simulink model "s_carro_pend"  (R2014a)
settings: Solver=ode3  StartTime=0.0  StopTime=inf  FixedStep=h  RelTol=1e-3
values from neighbouring files (symbols this model uses):
  g = 9.81    [Constantes.m]
  l = 0.641    [Constantes.m]
  m = 0.23    [Constantes.m]
  M = 0.57    [Constantes.m]
undefined symbols (not defined in the file or in its folder): br, bt
libraries: vrlib x3, fuzblock x1
settings Model: Creator=Jovani  LastModifiedBy=Lalo
settings OptimizationCC: SimCompilerOptimization=off
settings DebuggingCC: UnderspecifiedInitializationDetection=Classic  FrameProcessingCompatibilityMsg=error  StateNameClashWarn=warning
settings HardwareCC: ProdBitPerLong=64  ProdBitPerPointer=64  ProdIntDivRoundTo=Zero  ProdEndianess=LittleEndian  ProdWordSize=64  ProdHWDeviceType=Intel->x86-64  TargetBitPerLong=64  TargetBitPerPointer=64  TargetIntDivRoundTo=Zero  TargetEndianess=LittleEndian  TargetWordSize=64  TargetHWDeviceType=Intel->x86-64
settings RTWCC: SystemTargetFile=sldrt.tlc  TemplateMakefile=sldrt.tmf  Description=Simulink Desktop Real-Time  RTWCompilerOptimization=on
settings CodeAppCC: MaxIdLength=95
settings SimulinkDesktopRealTimeCC: TargetPreCompLibLocation=C:\Program Files\MATLAB\R2016a\toolbox\sldrt\lib\win64  TargetLangStandard=C89/C90 (ANSI)  SupportVariableSizeSignals=off
settings ConfigComp: CovMetricSettings=dw  CovHtmlReporting=on  CovSaveCumulativeToWorkspaceVar=on  CovSaveSingleToWorkspaceVar=on  CovModelRefEnable=Off  CovExternalEMLEnable=off

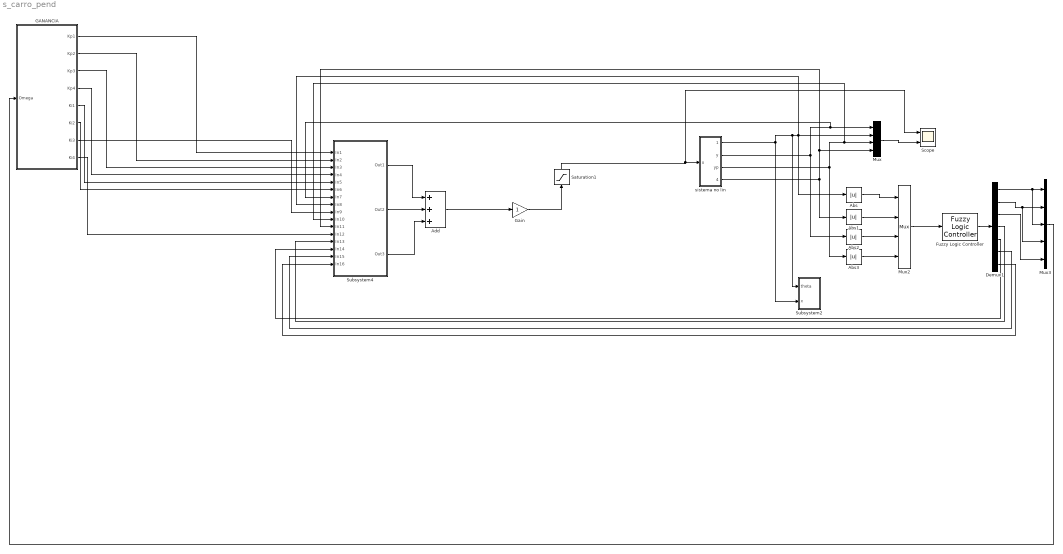
== system s_carro_pend ==
  Abs{,1..3} (4 alike) : Abs
  Add : Sum  Inputs=+++
  Demux1 : Demux  Outputs=7
  Fuzzy Logic Controller : fuzblock/Fuzzy Logic  Controller  fis=pi_2
  GANANCIA : Subsystem
  Gain : Gain
  Mux : Mux
  Mux2 : Mux
  Mux3 : Mux  Inputs=5
  Saturation1 : Saturate  UpperLimit=7.5  LowerLimit=-7.5
  Scope : Scope  NumInputPorts=2
      settings: YMin=-5~-5  YMax=5~5
  Subsystem2 : Subsystem
  Subsystem4 : Subsystem
  sistema no lin : Subsystem
  wires:
  Mux/1 -> Scope/2
  Gain/1 -> Saturation1/1
  Add/1 -> Gain/1
  sistema no lin/2(y) -> Abs2/1, Subsystem4/7(In7), Mux/1
  sistema no lin/3(yp) -> Abs3/1, Subsystem4/10(In10), Mux/3
  sistema no lin/1(theta) -> Subsystem2/2(x), Subsystem2/1(theta), Abs/1, Subsystem4/8(In8), Mux/2
  sistema no lin/4(thetap) -> Abs1/1, Subsystem4/11(In11), Mux/4
  Abs/1 -> Mux2/1
  Abs1/1 -> Mux2/2
  Abs2/1 -> Mux2/3
  Abs3/1 -> Mux2/4
  Mux2/1 -> Fuzzy Logic Controller/1
  Fuzzy Logic Controller/1 -> Demux1/1
  Demux1/1 -> Mux3/3, Mux3/1
  Demux1/2 -> Mux3/4, Mux3/2
  Demux1/3 -> Mux3/5
  Mux3/1 -> GANANCIA/1(Omega)
  Saturation1/1 -> Scope/1, sistema no lin/1("u ")
  ? -> ?
  GANANCIA/1(Kp1) -> Subsystem4/1(In1)
  GANANCIA/2(Kp2) -> Subsystem4/2(In2)
  GANANCIA/3("Kp3 ") -> Subsystem4/3(In3)
  GANANCIA/4(Kp4) -> Subsystem4/4(In4)
  GANANCIA/5("Ki1 ") -> Subsystem4/5(In5)
  GANANCIA/6("Ki2 ") -> Subsystem4/6(In6)
  GANANCIA/7("Ki3 ") -> Subsystem4/9(In9)
  GANANCIA/8("Ki4 ") -> Subsystem4/12(In12)
  Demux1/4 -> Subsystem4/13(In13)
  Demux1/5 -> Subsystem4/14(In14)
  Demux1/6 -> Subsystem4/15(In15)
  Demux1/7 -> Subsystem4/16(In16)
  Subsystem4/1(Out1) -> Add/1
  Subsystem4/2(Out2) -> Add/2
  Subsystem4/3(Out3) -> Add/3

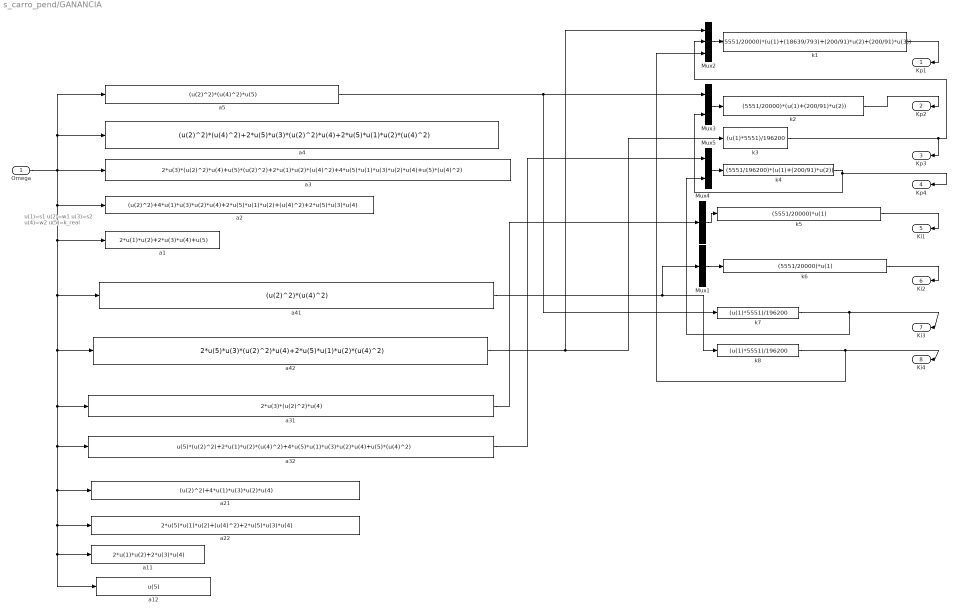
== system s_carro_pend/GANANCIA ==
  note: u(1)=s1
      | u(2)=w1
      | u(3)=s2
      | u(4)=w2
      | u(5)=k_real
  Omega : Inport
  Mux1 : Mux  Inputs=1
  Mux2 : Mux  Inputs=3
  Mux3 : Mux  Inputs=2
  Mux4 : Mux  Inputs=1
  Mux5 : Mux  Inputs=2
  "a1 " : Fcn  Expr=2*u(1)*u(2)+2*u(3)*u(4)+u(5)
  "a11 " : Fcn  Expr=2*u(1)*u(2)+2*u(3)*u(4)
  a12 : Fcn  Expr=u(5)
  "a2 " : Fcn  Expr=(u(2)^2)+4*u(1)*u(3)*u(2)*u(4)+2*u(5)*u(1)*u(2)+(u(4)^2)+2*u(5)*u(3)*u(4)
  "a21 " : Fcn  Expr=(u(2)^2)+4*u(1)*u(3)*u(2)*u(4)
  "a22 " : Fcn  Expr=2*u(5)*u(1)*u(2)+(u(4)^2)+2*u(5)*u(3)*u(4)
  a3 : Fcn  Expr=2*u(3)*(u(2)^2)*u(4)+u(5)*(u(2)^2)+2*u(1)*u(2)*(u(4)^2)+4*u(5)*u(1)*u(3)*u(2)*u(4)+u(5)*(u(4)^2)
  a31 : Fcn  Expr=2*u(3)*(u(2)^2)*u(4)
  a32 : Fcn  Expr=u(5)*(u(2)^2)+2*u(1)*u(2)*(u(4)^2)+4*u(5)*u(1)*u(3)*u(2)*u(4)+u(5)*(u(4)^2)
  a4 : Fcn  Expr=(u(2)^2)*(u(4)^2)+2*u(5)*u(3)*(u(2)^2)*u(4)+2*u(5)*u(1)*u(2)*(u(4)^2)
  a41 : Fcn  Expr=(u(2)^2)*(u(4)^2)
  a42 : Fcn  Expr=2*u(5)*u(3)*(u(2)^2)*u(4)+2*u(5)*u(1)*u(2)*(u(4)^2)
  a5 : Fcn  Expr=(u(2)^2)*(u(4)^2)*u(5)
  k1 : Fcn  Expr=(5551/20000)*(u(1)+(18639/793)+(200/91)*u(2)+(200/91)*u(3))
  k2 : Fcn  Expr=(5551/20000)*(u(1)+(200/91)*u(2))
  k3 : Fcn  Expr=(u(1)*5551)/196200
  k4 : Fcn  Expr=(5551/196200)*(u(1)+(200/91)*u(2))
  "k5 " : Fcn  Expr=(5551/20000)*u(1)
  "k6 " : Fcn  Expr=(5551/20000)*u(1)
  k7 : Fcn  Expr=(u(1)*5551)/196200
  k8 : Fcn  Expr=(u(1)*5551)/196200
  Kp1 : Outport
  Kp2 : Outport  Port=2
  "Kp3 " : Outport  Port=3
  Kp4 : Outport  Port=4
  "Ki1 " : Outport  Port=5
  "Ki2 " : Outport  Port=6
  "Ki3 " : Outport  Port=7
  "Ki4 " : Outport  Port=8
  wires:
  a32/1 -> Mux5/1
  Mux5/1 -> k4/1
  Mux1/1 -> "k6 "/1
  "k6 "/1 -> "Ki2 "/1
  a31/1 -> Mux4/1
  a41/1 -> k8/1, Mux1/1
  a42/1 -> k3/1, Mux2/1
  k2/1 -> Kp2/1
  k1/1 -> Kp1/1
  Mux3/1 -> k2/1
  Mux2/1 -> k1/1
  k4/1 -> Kp4/1, Mux3/2
  "k5 "/1 -> "Ki1 "/1
  k8/1 -> "Ki4 "/1, Mux2/3
  k3/1 -> "Kp3 "/1, Mux2/2
  a5/1 -> Mux3/1, k7/1
  k7/1 -> "Ki3 "/1, Mux5/2
  Omega/1 -> a4/1, a5/1, a3/1, "a2 "/1, "a1 "/1, a41/1, a42/1, a31/1, a32/1, "a21 "/1, "a22 "/1, "a11 "/1, a12/1
  Mux4/1 -> "k5 "/1

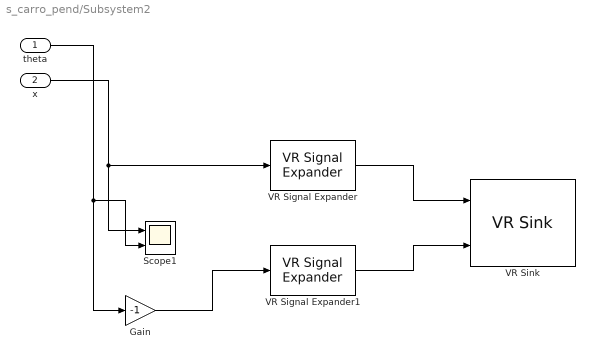
== system s_carro_pend/Subsystem2 ==
  theta : Inport
  x : Inport  Port=2
  Gain : Gain  Gain=-1
  Scope1 : Scope  NumInputPorts=2
      settings: YMin=3.51931e+09~-5.59031e+09  YMax=3.51951e+09~-5.5902e+09
  VR Signal Expander : vrlib/VR Signal Expander  outwidth=3  outidx=[1]
  VR Signal Expander1 : vrlib/VR Signal Expander  outwidth=4  outidx=[4]
  VR Sink : vrlib/VR Sink  InstantiateOnLoad=on  SampleTime=0.1  ViewEnable=on  RemoteChange=off  RemoteView=off  FieldsWritten=Carro.rotation.4.1.1.double#Carro.translation.3.1.1.double  WorldFileName=C:\Users\Lalo\Desktop\MC Automatizacion\Segundo Semestre\Control Int\Carro_pendulo\pendulo_invertido.wrl  AutoView=off  VideoDimensions=[]  AllowVariableSize=off
  wires:
  Gain/1 -> VR Signal Expander1/1
  x/1 -> Scope1/1, VR Signal Expander/1
  theta/1 -> Gain/1, Scope1/2
  VR Signal Expander/1 -> VR Sink/1
  VR Signal Expander1/1 -> VR Sink/2

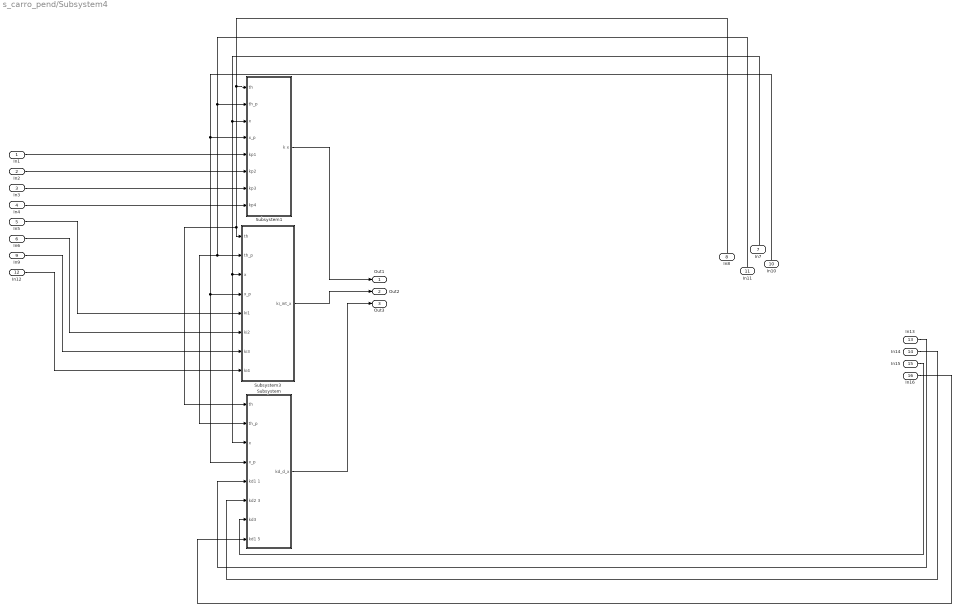
== system s_carro_pend/Subsystem4 ==
  In1 : Inport
  In2 : Inport  Port=2
  In3 : Inport  Port=3
  In4 : Inport  Port=4
  In5 : Inport  Port=5
  In6 : Inport  Port=6
  In7 : Inport  Port=7
  In8 : Inport  Port=8
  In9 : Inport  Port=9
  In10 : Inport  Port=10
  In11 : Inport  Port=11
  In12 : Inport  Port=12
  In13 : Inport  Port=13
  In14 : Inport  Port=14
  In15 : Inport  Port=15
  In16 : Inport  Port=16
  Subsystem : Subsystem
  Subsystem1 : Subsystem
  Subsystem3 : Subsystem
  Out1 : Outport
  Out2 : Outport  Port=2
  Out3 : Outport  Port=3
  wires:
  In1/1 -> Subsystem1/5("kp1 ")
  In2/1 -> Subsystem1/6(kp2)
  In3/1 -> Subsystem1/7(kp3)
  In4/1 -> Subsystem1/8(kp4)
  In5/1 -> Subsystem3/5(ki1)
  In6/1 -> Subsystem3/6(ki2)
  In9/1 -> Subsystem3/7(ki3)
  In12/1 -> Subsystem3/8(ki4)
  Subsystem1/1(k x) -> Out1/1
  Subsystem3/1(ki_int_x) -> Out2/1
  Subsystem/1("kd_d_x ") -> Out3/1
  In13/1 -> Subsystem/5(kd1 1)
  In14/1 -> Subsystem/6(kd2 3)
  In15/1 -> Subsystem/7("kd3 ")
  In16/1 -> Subsystem/8(kd1 5)
  In10/1 -> Subsystem/4("x_p "), Subsystem3/4(x_p), Subsystem1/4(x_p)
  In11/1 -> Subsystem/2("th_p "), Subsystem3/2(th_p), Subsystem1/2(th_p)
  In8/1 -> Subsystem1/1("th "), Subsystem/1("th "), Subsystem3/1("th ")
  In7/1 -> Subsystem/3("x "), Subsystem3/3(x), Subsystem1/3(x)

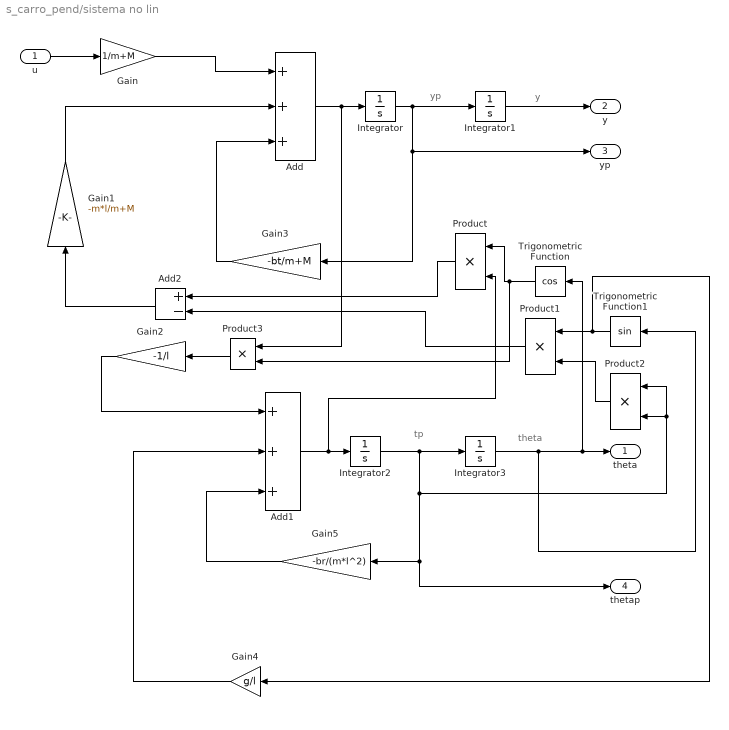
== system s_carro_pend/sistema no lin ==
  note: yp
  note: y
  note: tp
  note: theta
  "u " : Inport
  Add : Sum  Inputs=+++
  Add1 : Sum  Inputs=+++
  Add2 : Sum  Inputs=+-
  Gain : Gain  Gain=1/m+M
  Gain1 : Gain  Gain=-m*l/m+M
  Gain2 : Gain  Gain=-1/l
  Gain3 : Gain  Gain=-bt/m+M
  Gain4 : Gain  Gain=g/l
  Gain5 : Gain  Gain=-br/(m*l^2)
  Integrator : Integrator
  Integrator1 : Integrator
  Integrator2 : Integrator
  Integrator3 : Integrator  InitialCondition=0.1
  Product{,1..3} (4 alike) : Product
  Trigonometric Function : Trigonometry  Operator=cos
  Trigonometric Function1 : Trigonometry
  theta : Outport
  y : Outport  Port=2
  yp : Outport  Port=3
  thetap : Outport  Port=4
  wires:
  Gain5/1 -> Add1/3
  Add1/1 -> Product/2, Integrator2/1
  Gain/1 -> Add/1
  Integrator3/1 -> Trigonometric Function1/1, Trigonometric Function/1, theta/1
  Integrator2/1 -> Integrator3/1, thetap/1, Gain5/1, Product2/1, Product2/2
  Gain4/1 -> Add1/2
  Integrator/1 -> yp/1, Gain3/1, Integrator1/1
  Integrator1/1 -> y/1
  Gain3/1 -> Add/3
  Add/1 -> Integrator/1, Product3/1
  Gain2/1 -> Add1/1
  "u "/1 -> Gain/1
  Gain1/1 -> Add/2
  Trigonometric Function/1 -> Product3/2, Product/1
  Product/1 -> Add2/1
  Add2/1 -> Gain1/1
  Trigonometric Function1/1 -> Gain4/1, Product1/1
  Product1/1 -> Add2/2
  Product2/1 -> Product1/2
  Product3/1 -> Gain2/1

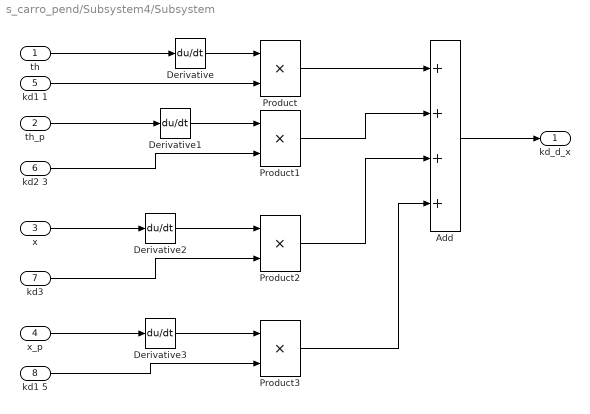
== system s_carro_pend/Subsystem4/Subsystem ==
  "th " : Inport
  "th_p " : Inport  Port=2
  "x " : Inport  Port=3
  "x_p " : Inport  Port=4
  kd1 1 : Inport  Port=5
  kd2 3 : Inport  Port=6
  "kd3 " : Inport  Port=7
  kd1 5 : Inport  Port=8
  Add : Sum  Inputs=++++
  Derivative{,1..3} (4 alike) : Derivative
  Product{,1..3} (4 alike) : Product
  "kd_d_x " : Outport
  wires:
  Derivative/1 -> Product/1
  Derivative1/1 -> Product1/1
  Product2/1 -> Add/3
  kd1 1/1 -> Product/2
  Product3/1 -> Add/4
  Product1/1 -> Add/2
  Add/1 -> "kd_d_x "/1
  kd1 5/1 -> Product3/2
  kd2 3/1 -> Product1/2
  Derivative3/1 -> Product3/1
  Product/1 -> Add/1
  "x "/1 -> Derivative2/1
  "x_p "/1 -> Derivative3/1
  "th_p "/1 -> Derivative1/1
  Derivative2/1 -> Product2/1
  "kd3 "/1 -> Product2/2
  "th "/1 -> Derivative/1

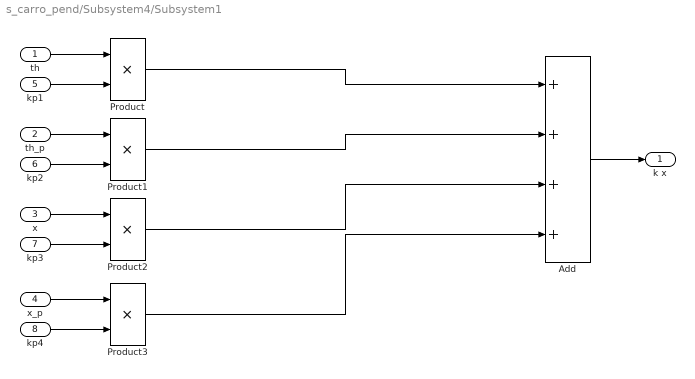
== system s_carro_pend/Subsystem4/Subsystem1 ==
  "th " : Inport
  th_p : Inport  Port=2
  x : Inport  Port=3
  x_p : Inport  Port=4
  "kp1 " : Inport  Port=5
  kp2 : Inport  Port=6
  kp3 : Inport  Port=7
  kp4 : Inport  Port=8
  Add : Sum  Inputs=++++
  Product{,1..3} (4 alike) : Product
  k x : Outport
  wires:
  th_p/1 -> Product1/1
  "th "/1 -> Product/1
  x/1 -> Product2/1
  "kp1 "/1 -> Product/2
  kp4/1 -> Product3/2
  Product2/1 -> Add/3
  x_p/1 -> Product3/1
  Product3/1 -> Add/4
  kp2/1 -> Product1/2
  kp3/1 -> Product2/2
  Add/1 -> k x/1
  Product/1 -> Add/1
  Product1/1 -> Add/2

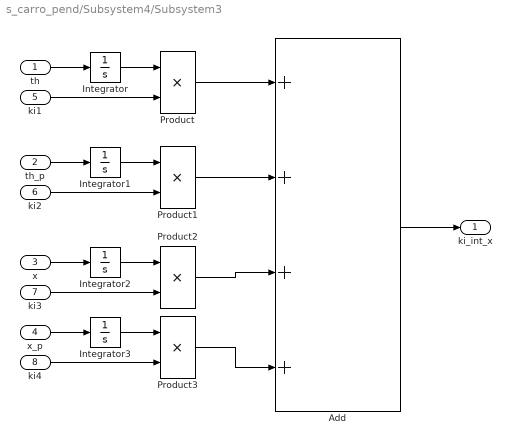
== system s_carro_pend/Subsystem4/Subsystem3 ==
  "th " : Inport
  th_p : Inport  Port=2
  x : Inport  Port=3
  x_p : Inport  Port=4
  ki1 : Inport  Port=5
  ki2 : Inport  Port=6
  ki3 : Inport  Port=7
  ki4 : Inport  Port=8
  Add : Sum  Inputs=++++
  Integrator{,1..3} (4 alike) : Integrator
  Product{,1..3} (4 alike) : Product
  ki_int_x : Outport
  wires:
  Product3/1 -> Add/4
  Product2/1 -> Add/3
  Product/1 -> Add/1
  Integrator3/1 -> Product3/1
  "th "/1 -> Integrator/1
  ki1/1 -> Product/2
  ki2/1 -> Product1/2
  ki3/1 -> Product2/2
  ki4/1 -> Product3/2
  Product1/1 -> Add/2
  th_p/1 -> Integrator1/1
  Integrator1/1 -> Product1/1
  x_p/1 -> Integrator3/1
  Integrator2/1 -> Product2/1
  x/1 -> Integrator2/1
  Integrator/1 -> Product/1
  Add/1 -> ki_int_x/1

== matlab function s_carro_pend/MATLAB Function1 ==
  data: R input; kf output
function kf = fcn(R)
%#codegen
%kf=[-60.1155,-15.6512,-6.3246,-10.4452];
kf=[-60.1155,-15.6512,-6.3246,-10.4452];

end
